simulink model "fmcw_range_model"  (R2024b)
settings: Solver=FixedStepDiscrete  StartTime=0.0  StopTime=10e-6  FixedStep=5e-9  RelTol=1e-3
undefined symbols (not defined in the file or in its folder): physconst
libraries: phasedenvlib x3, phasedtxrxlib x3, phaseddetectlib x1, phasedwavlib x1, phaseddoalib x1
settings Model: Creator=lloyd  LastModifiedBy=lloyd

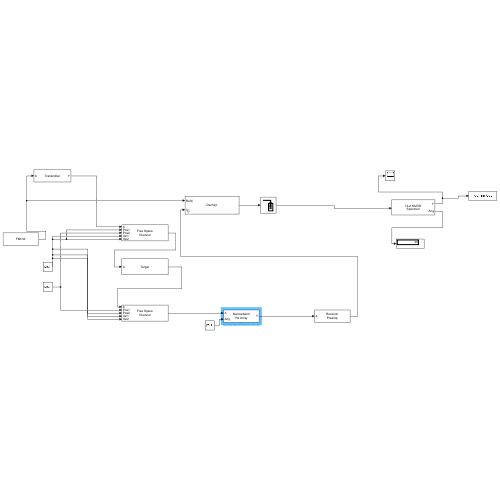
[thumbnail: Simulink's stored preview of the top-level diagram]
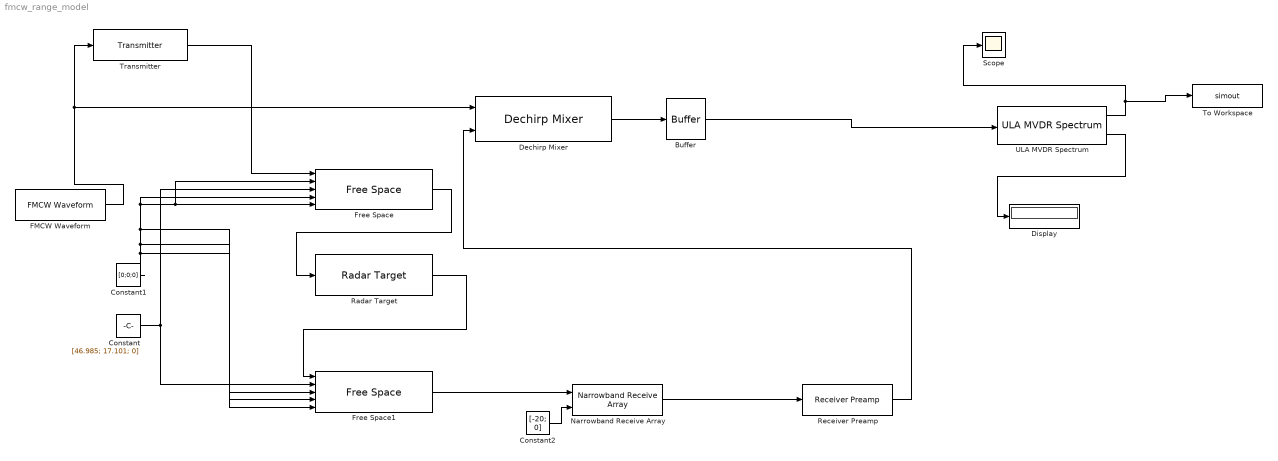
== system fmcw_range_model ==
  Buffer : Buffer  N=2000  OutputFrames=off
  Constant : Constant  Value=[46.985; 17.101; 0]
  Constant1 : Constant  Value=[0;0;0]
  Constant2 : Constant  Value=[-20; 0]
  Dechirp Mixer : phaseddetectlib/Dechirp Mixer
  Display : Display
  FMCW Waveform : phasedwavlib/FMCW Waveform  SampleRate=200e6  SweepTime=10e-6  SweepBandwidth=150e6  SweepDirection=Up  SweepInterval=Positive  OutputFormat=Samples  NumSamples=100  NumSweeps=1  SimulateUsing=Interpreted execution
  Free Space : phasedenvlib/Free Space  PropagationSpeed=3e8  OperatingFrequency=77e9  TwoWayPropagation=off  SampleRateFromInputCheckbox=on  SampleRate=1e6  MaximumDistanceSource=Property  MaximumDistance=500  MaximumNumInputSamplesSource=Auto  MaximumNumInputSamples=1000  SimulateUsing=Interpreted execution
  Free Space1 : phasedenvlib/Free Space  PropagationSpeed=3e8  OperatingFrequency=77e9  TwoWayPropagation=off  SampleRateFromInputCheckbox=on  SampleRate=1e6  MaximumDistanceSource=Property  MaximumDistance=500  MaximumNumInputSamplesSource=Auto  MaximumNumInputSamples=1000  SimulateUsing=Interpreted execution
  Narrowband Receive Array : phasedtxrxlib/Narrowband Receive Array  PropagationSpeed=physconst( 'LightSpeed' )  OperatingFrequency=77e9  Wavefront=Plane  SensorGainMeasure=dB  Polarization=None  WeightsInputPort=off  SimulateUsing=Interpreted execution  Sensor=phased.ULA(Element=phased.IsotropicAntennaElement(FrequencyRange=[76.925e9 77.075e9]),NumElements=8,ElementSpacing=1.948e-3)
  Radar Target : phasedenvlib/Radar Target  EnablePolarization=off  Mode=Monostatic  MeanRCSSource=Property  ScatteringMatrixSource=Property  MeanRCS=10  ScatteringMatrix=eye( 2 )  Model=Nonfluctuating  PropagationSpeed=physconst( 'LightSpeed' )  OperatingFrequency=77e9  SeedSource=Auto  Seed=0  SimulateUsing=Interpreted execution
  Receiver Preamp : phasedtxrxlib/Receiver Preamp  Gain=0  LossFactor=0  NoiseMethod=Noise temperature  NoiseFigure=3  ReferenceTemperature=290  SampleRateFromInputCheckbox=on  SampleRate=1e6  NoisePower=0  EnableInputPort=off  PhaseNoiseInputPort=off  SeedSource=Auto  Seed=0  SimulateUsing=Interpreted execution
  Scope : Scope
  To Workspace : ToWorkspace  VariableName=simout  SaveFormat=Timeseries  SampleTime=-1
  Transmitter : phasedtxrxlib/Transmitter  PeakPower=1  GainMethod=Linear  Gain=120  LossFactor=0  OIP3=Inf  Table=[ -25, 5, -1; -10, 20, -2; 0, 27, 12; 5, 28, 12 ]  InUseOutputPort=off  CoherentOnTransmit=on  PhaseNoiseOutputPort=off  SimulateUsing=Interpreted execution  NoiseMethod=None  NoiseFigure=3  NoiseFactor=2  NoiseTemperature=290  ReferenceTemperature=290  SampleRate=1e6  SampleRateFromInputCheckbox=on  PhaseOffset=0  SeedSource=Auto  Seed=0
  ULA MVDR Spectrum : phaseddoalib/ULA MVDR Spectrum  PropagationSpeed=physconst( 'LightSpeed' )  OperatingFrequency=77e9  NumPhaseShifterBits=0  ForwardBackwardAveraging=off  SpatialSmoothing=0  ScanAngles=-90:0.5:90  DOAOutputPort=on  NumSignals=1  SimulateUsing=Interpreted execution  SensorArray=phased.ULA(Element=phased.IsotropicAntennaElement(FrequencyRange=[76.925e9 77.075e9]),NumElements=8,ElementSpacing=1.9481e-3)
  wires:
  Constant1/1 -> Free Space1/3, Free Space1/4, Free Space/4, Free Space/2, Free Space/5, Free Space1/5
  Constant/1 -> Free Space/3, Free Space1/2
  Free Space/1 -> Radar Target/1
  Dechirp Mixer/1 -> Buffer/1
  Radar Target/1 -> Free Space1/1
  Free Space1/1 -> Narrowband Receive Array/1
  Constant2/1 -> Narrowband Receive Array/2
  ULA MVDR Spectrum/2 -> Display/1
  ULA MVDR Spectrum/1 -> To Workspace/1, Scope/1
  Narrowband Receive Array/1 -> Receiver Preamp/1
  Receiver Preamp/1 -> Dechirp Mixer/2
  Buffer/1 -> ULA MVDR Spectrum/1
  FMCW Waveform/1 -> Dechirp Mixer/1, Transmitter/1
  Transmitter/1 -> Free Space/1
